simulink model "state_space_last_figure"  (Simulink 7.5)
settings: Solver=ode45  StartTime=0.0  StopTime=10.0  RelTol=1e-3
values from neighbouring files (symbols this model uses):
  b1 = 500    [initialise_parameters.m]
  b2 = 1500    [initialise_parameters.m]
  k1 = 60000*4    (= 240000)    [initialise_parameters.m]
  k2 = 1350000*4    (= 5400000)    [initialise_parameters.m]
  m1 = 500    [initialise_parameters.m]
  m2 = 50    [initialise_parameters.m]
settings Model: Creator=Arijit  LastModifiedBy=Arijit

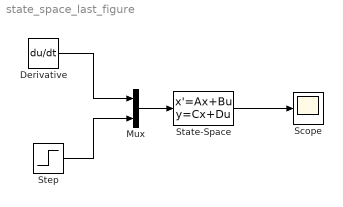
== system state_space_last_figure ==
  Derivative : Derivative
  Mux : Mux  Inputs=2
  Scope : Scope
  State-Space : StateSpace  A=[-b1/m1 b1/m1 -k1/m1 k1/m1; b1/m1 -(b1+b2)/m2 k1/m1 -(k1+k2)/m2;1 0 0 0; 0 1 0 0]  B=[0 0; b2/m2 k2/m2;0 0;0 0]  C=[0 0 1 0; 0 0 0 1; 0 0 1 -1]  D=[0 0;0 0;0 0]
  Step : Step  SampleTime=0
  wires:
  Derivative/1 -> Mux/1
  Step/1 -> Mux/2
  Mux/1 -> State-Space/1
  State-Space/1 -> Scope/1
